simulink model "x_controller_sim"  (R2020b)
settings: Solver=VariableStepAuto  StartTime=0.0  StopTime=10  RelTol=1e-3
values from neighbouring files (symbols this model uses):
  b = 3.5077E-6    (= 3.5077e-06)    [x_controller_script.m]
  J = 3.2284E-6    (= 3.2284e-06)    [x_controller_script.m]
  Kb = 0.0274    [x_controller_script.m]
  Kt = 0.0274    [x_controller_script.m]
  L = 2.75E-6    (= 2.75e-06)    [x_controller_script.m]
  R = 4    [x_controller_script.m]
  theta = 180    [x_controller_script.m]
settings Model: PacingRate=0.350000  Creator=onepunchass  LastModifiedBy=onepunchass

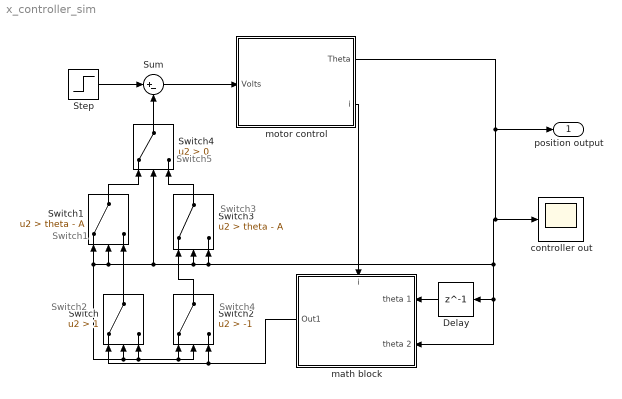
== system x_controller_sim ==
  note: Switch5
  note: Switch4
  note: Switch2
  note: Switch3
  note: Switch1
  Delay : Delay  DelayLength=1  InitialCondition=0
  Step : Step  After=theta  SampleTime=0
  Sum : Sum  Inputs=|+-
  Switch : Switch  Criteria=u2 > Threshold  Threshold=1
  Switch1 : Switch  Criteria=u2 > Threshold  Threshold=theta - A  ZeroCross=off
  Switch2 : Switch  Criteria=u2 > Threshold  Threshold=-1
  Switch3 : Switch  Criteria=u2 > Threshold  Threshold=theta - A  ZeroCross=off
  Switch4 : Switch  Criteria=u2 > Threshold  ZeroCross=off
  controller out : Scope
  math block : Subsystem
      settings: PortSchema="{\"entries\":[{\"content\":{\"sides\":[{\"content\":{\"connectorIds\":[\"Out1\"]},\"type\":\"ConnectorPlacement.EquallySpacedRectSide\",\"uuid\":\"7b2525ee-f4b3-4012-96d8-73c23f64b492\"},{\"content\":{\"connectorIds\":[\"In2\",\"In3\"],\"side\":\"RIGHT\"},\"type\":\"ConnectorPlacement.EquallySpacedRectSide\",\"uuid\":\"d5f03473-39b5-4853-a461-ee9452a01372\"},{\"content\":{\"connectorIds\":[\"In1\"],\"side\":\"TOP\"},\"type\":\"ConnectorPlacement.EquallySpacedRectSide\",\"uuid\":\"e823bf3c-e89a-43b1-9e18-8b6c20d83bd9\"},{\"content\":{\"connectorIds\":[],\"side\":\"HIDDEN\"},\"type\":\"ConnectorPlacement.EquallySpacedRectSide\",\"uuid\":\"a155a483-97d5-4c2f-b6f2-77a4b24376a6\"}]},\"type\":\"ConnectorPlacement.EquallySpacedConnector\",\"uuid\":\"2c2a0c64-272f-44ce-a143-7e1c11e05d61\"}],\"packageUris\":[\"http://schema.mathworks.com/mf0/Connector/R2020b\"],\"version\":\"1.0\"}"
  motor control : Subsystem
  position output : Outport
  wires:
  Step/1 -> Sum/1
  Delay/1 -> math block/2(theta 1)
  motor control/2(i) -> math block/1(i)
  math block/1(Out1) -> Switch2/3, Switch/1
  motor control/1(Theta) -> math block/3(theta 2), Delay/1, Switch4/2, Switch2/2, Switch2/1, Switch/3, Switch/2, Switch1/1, Switch1/2, Switch3/2, Switch3/3, controller out/1, position output/1
  Switch/1 -> Switch1/3
  Sum/1 -> motor control/1(Volts)
  Switch2/1 -> Switch3/1
  Switch4/1 -> Sum/2
  Switch1/1 -> Switch4/1
  Switch3/1 -> Switch4/3

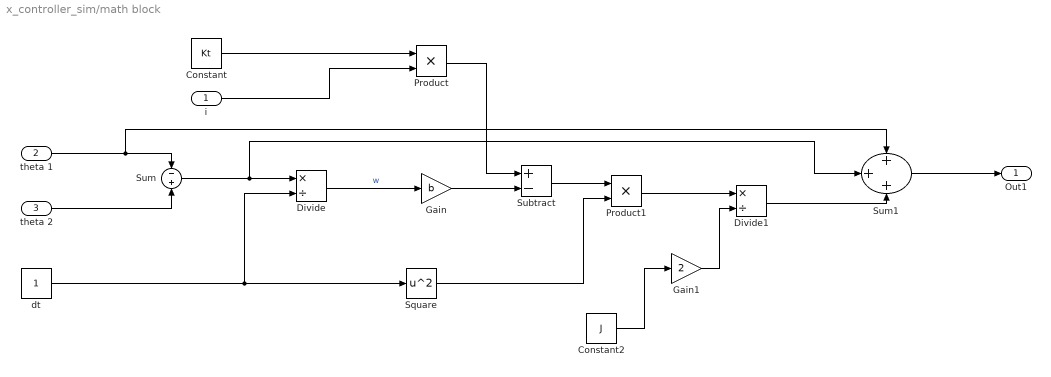
== system x_controller_sim/math block ==
  i : Inport
  theta 1 : Inport  Port=2
  theta 2 : Inport  Port=3
  Constant : Constant  Value=Kt
  Constant2 : Constant  Value=J
  Divide : Product  Inputs=*/
  Divide1 : Product  Inputs=*/
  Gain : Gain  Gain=b
  Gain1 : Gain  Gain=2
  Product : Product
  Product1 : Product
  Square : Math  Operator=square  SaturateOnIntegerOverflow=on
  Subtract : Sum  Inputs=+-
  Sum : Sum  Inputs=-+
  Sum1 : Sum  Inputs=+++
  dt : Constant
  Out1 : Outport
  wires:
  theta 2/1 -> Sum/2
  theta 1/1 -> Sum1/1, Sum/1
  dt/1 -> Square/1, Divide/2
  Sum/1 -> Sum1/2, Divide/1
  Divide/1 -> Gain/1  "w"
  Gain/1 -> Subtract/2
  Constant/1 -> Product/1
  i/1 -> Product/2
  Product/1 -> Subtract/1
  Subtract/1 -> Product1/1
  Square/1 -> Product1/2
  Product1/1 -> Divide1/1
  Constant2/1 -> Gain1/1
  Gain1/1 -> Divide1/2
  Sum1/1 -> Out1/1
  Divide1/1 -> Sum1/3

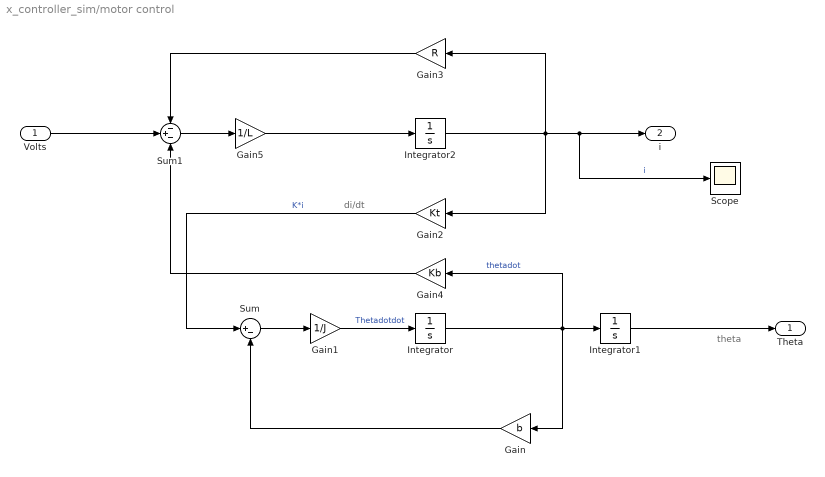
== system x_controller_sim/motor control ==
  note: di/dt
  note: theta
  Volts : Inport
  Gain : Gain  Gain=b
  Gain1 : Gain  Gain=1/J
  Gain2 : Gain  Gain=Kt
  Gain3 : Gain  Gain=R
  Gain4 : Gain  Gain=Kb
  Gain5 : Gain  Gain=1/L
  Integrator : Integrator
  Integrator1 : Integrator
  Integrator2 : Integrator
  Scope : Scope
  Sum : Sum  Inputs=|+-
  Sum1 : Sum  Inputs=-+-
  Theta : Outport
  i : Outport  Port=2
  wires:
  Gain/1 -> Sum/2
  Gain5/1 -> Integrator2/1
  Integrator2/1 -> Scope/1, i/1, Gain3/1, Gain2/1  "i"
  Sum/1 -> Gain1/1
  Gain3/1 -> Sum1/1
  Gain2/1 -> Sum/1  "K*i"
  Volts/1 -> Sum1/2
  Gain4/1 -> Sum1/3
  Sum1/1 -> Gain5/1
  Gain1/1 -> Integrator/1  "Thetadotdot"
  Integrator1/1 -> Theta/1
  Integrator/1 -> Gain4/1, Gain/1, Integrator1/1  "thetadot"
